simulink model "networkanalyzer"  (R2012b)
settings: Solver=ode3  SolverMode=SingleTasking  StartTime=0.0  StopTime=50000  RelTol=1e-3
libraries: xbsIndex_r4 x1097, casper_library_flow_control x33, casper_library_misc x21, xps_library x10
(part 3 of 8)

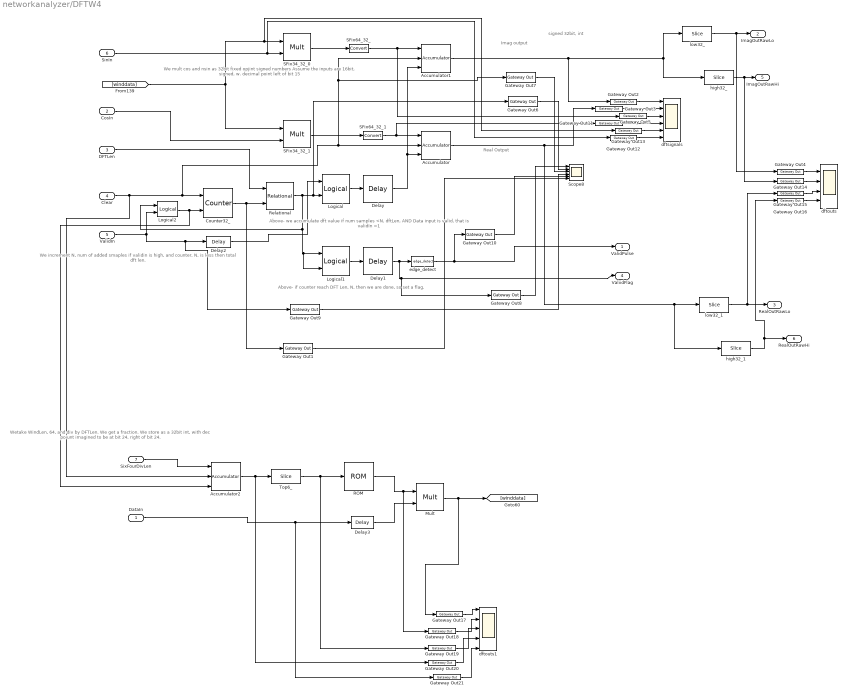
== system networkanalyzer/DFTW4 ==
  note: Wetake WindLen, 64, and div by DFTLen.
      | We get a fraction. We store as a 32bit int, with dec poiunt imagined to
      | be at bit 24, right of bit 24.
  note: Real Output
  note: Imag output
  note: We mult cos and nsin as 32bit fixed opjint signed numbers
      | Assume the inputs are 16bit, signed, w. decimal point left of bit 15
  note: Above- if counter reach DFT Len, N, then we are done, so set a flag.
  note: Above- we accumulate dft value if num samples <N, dftLen, AND
      | Data input is valid, that is validIn =1
  note: We increment N, num of added smaples if validin is high, and
      | counter, N, is less then total dft len.
  note: signed 32bit, int
  DataIn : Inport
  CosIn : Inport  Port=2
  DFTLen : Inport  Port=3
  Clear : Inport  Port=4
  ValidIn : Inport  Port=5
  SinIn : Inport  Port=6
  SixFourDivLen : Inport  Port=7
  Accumulator : xbsIndex_r4/Accumulator  operation=Add  n_bits=64  overflow=Wrap  scale=1  rst=on  hasbypass=off  en=on  dbl_ovrd=off  use_behavioral_HDL=on  implementation=Fabric  block_type=accum
  Accumulator1 : xbsIndex_r4/Accumulator  operation=Add  n_bits=64  overflow=Wrap  scale=1  rst=on  hasbypass=off  en=on  dbl_ovrd=off  use_behavioral_HDL=on  implementation=Fabric  block_type=accum
  Accumulator2 : xbsIndex_r4/Accumulator  operation=Add  n_bits=32  overflow=Wrap  scale=1  rst=on  hasbypass=off  en=on  dbl_ovrd=off  use_behavioral_HDL=on  implementation=Fabric  block_type=accum
  Counter32_ : xbsIndex_r4/Counter  cnt_type=Free Running  cnt_to=Inf  operation=Up  start_count=0  cnt_by_val=1  arith_type=Unsigned  n_bits=32  bin_pt=0  load_pin=off  rst=on  en=on  explicit_period=on  period=1  dbl_ovrd=off  use_behavioral_HDL=off  implementation=Fabric  block_type=counter
  Delay : xbsIndex_r4/Delay  rst=off  infoeditControl=Selection of Reset will increase slice count due to use of real FFs and instead of SRLs  en=off  latency=2  dbl_ovrd=off  reg_retiming=off  block_type=delay
  Delay1 : xbsIndex_r4/Delay  rst=off  infoeditControl=Selection of Reset will increase slice count due to use of real FFs and instead of SRLs  en=off  latency=2  dbl_ovrd=off  reg_retiming=off  block_type=delay
  Delay2 : xbsIndex_r4/Delay  rst=off  infoeditControl=Selection of Reset will increase slice count due to use of real FFs and instead of SRLs  en=off  latency=2  dbl_ovrd=off  reg_retiming=off  block_type=delay
  Delay3 : xbsIndex_r4/Delay  rst=off  infoeditControl=Selection of Reset will increase slice count due to use of real FFs and instead of SRLs  en=off  latency=1  dbl_ovrd=off  reg_retiming=off  block_type=delay
  Gateway Out{1..21} (21 alike) : xbsIndex_r4/Gateway Out  inherit_from_input=off  hdl_port=off  timing_constraint=None  locs_specified=off  LOCs={}  UseAsDAC=off  DACChannel='1'  block_type=gatewayout
  Logical : xbsIndex_r4/Logical  logical_function=AND  inputs=2  en=off  latency=1  precision=Full  arith_type=Unsigned  n_bits=16  bin_pt=0  align_bp=on  dbl_ovrd=off  block_type=logical
  Logical1 : xbsIndex_r4/Logical  logical_function=NAND  inputs=2  en=off  latency=1  precision=Full  arith_type=Unsigned  n_bits=16  bin_pt=0  align_bp=on  dbl_ovrd=off  block_type=logical
  Logical2 : xbsIndex_r4/Logical  logical_function=AND  inputs=2  en=off  latency=0  precision=Full  arith_type=Unsigned  n_bits=16  bin_pt=0  align_bp=on  dbl_ovrd=off  block_type=logical
  Mult : xbsIndex_r4/Mult  precision=User Defined  arith_type="Signed  (2's comp)"  n_bits=16  bin_pt=15  quantization=Truncate  overflow=Wrap  en=off  latency=3  dbl_ovrd=off  use_behavioral_HDL=off  opt=Speed  use_embedded=on  optimum_pipeline=off  pipeline=on  use_rpm=on  placement_style=Triangular  block_type=mult
  ROM : xbsIndex_r4/ROM  depth=64  initVector=0.5-0.5*cos(2*pi*(0:63)/63)  distributed_mem=Block RAM  rst=off  init_reg=0  en=off  latency=1  gui_display_data_type=Fixed-point  arith_type="Signed  (2's comp)"  n_bits=16  bin_pt=15  preci_type=Single  exp_width=8  frac_width=24  dbl_ovrd=off  optimize=Area  use_rpm=on  block_type=sprom
  Relational : xbsIndex_r4/Relational  mode=a>=b  en=off  latency=1  dbl_ovrd=off  block_type=relational
  SFix34_32_0 : xbsIndex_r4/Mult  precision=User Defined  arith_type="Signed  (2's comp)"  n_bits=34  bin_pt=32  quantization=Truncate  overflow=Saturate  en=off  latency=4  dbl_ovrd=off  use_behavioral_HDL=off  opt=Speed  use_embedded=on  optimum_pipeline=off  pipeline=on  use_rpm=on  placement_style=Triangular  block_type=mult
  SFix34_32_1 : xbsIndex_r4/Mult  precision=User Defined  arith_type="Signed  (2's comp)"  n_bits=34  bin_pt=32  quantization=Truncate  overflow=Saturate  en=off  latency=4  dbl_ovrd=off  use_behavioral_HDL=off  opt=Speed  use_embedded=on  optimum_pipeline=off  pipeline=on  use_rpm=on  placement_style=Triangular  block_type=mult
  SFix64_32_ : xbsIndex_r4/Convert  gui_display_data_type=Fixed-point  arith_type="Signed  (2's comp)"  n_bits=64  bin_pt=32  float_type=Single  exp_bits=8  fraction_bits=24  quantization=Truncate  overflow=Wrap  en=off  latency=0  dbl_ovrd=off  pipeline=off  block_type=convert
  SFix64_32_1 : xbsIndex_r4/Convert  gui_display_data_type=Fixed-point  arith_type="Signed  (2's comp)"  n_bits=64  bin_pt=32  float_type=Single  exp_bits=8  fraction_bits=24  quantization=Truncate  overflow=Wrap  en=off  latency=0  dbl_ovrd=off  pipeline=off  block_type=convert
  Scope8 : Scope  NumInputPorts=6
      settings: YMin=0~-5~-5~-5~-5~-5  YMax=300000~5~5~5~5~5  SaveName=ScopeData18  MaxDataPoints=10000
  Top6_ : xbsIndex_r4/Slice  nbits=6  boolean_output=off  mode=Upper Bit Location + Width  bit1=0  base1=MSB of Input  bit0=0  base0=LSB of Input  dbl_ovrd=off  block_type=slice
  dftouts : Scope  NumInputPorts=4
      settings: YMin=0~-5~-5~-5  YMax=300000~5~5~5  SaveName=ScopeData5  MaxDataPoints=10000
  dftouts1 : Scope  NumInputPorts=5
      settings: YMin=-1~0~0~0~-1  YMax=5.55112e-17~1~70~5e+09~0  MaxDataPoints=10000
  dftsignals : Scope  NumInputPorts=6
      settings: YMin=0~-5~-5~-5~-5~-5  YMax=300000~5~5~5~5~5  SaveName=ScopeData4  MaxDataPoints=10000
  edge_detect : casper_library_misc/edge_detect  edge=Rising  polarity=Active High  x_in=[0 0.08 0.08 0.16 0.16 0.24 0.24 0.32 0.32 0.4]  y_in="[-1 -1  1  1  1  1  1  1  1  1]"  x_out=[0.6 0.68 0.68 0.76 0.76 0.84 0.84 0.92 0.92 1]  y_out="[-1 -1  1  1 -1 -1 -1 -1 -1 -1]"
  high32_ : xbsIndex_r4/Slice  nbits=32  boolean_output=off  mode=Lower Bit Location + Width  bit1=-32  base1=MSB of Input  bit0=32  base0=LSB of Input  dbl_ovrd=off  block_type=slice
  high32_1 : xbsIndex_r4/Slice  nbits=32  boolean_output=off  mode=Lower Bit Location + Width  bit1=-31  base1=MSB of Input  bit0=32  base0=LSB of Input  dbl_ovrd=off  block_type=slice
  low32_ : xbsIndex_r4/Slice  nbits=32  boolean_output=off  mode=Lower Bit Location + Width  bit1=-31  base1=MSB of Input  bit0=0  base0=LSB of Input  dbl_ovrd=off  block_type=slice
  low32_1 : xbsIndex_r4/Slice  nbits=32  boolean_output=off  mode=Lower Bit Location + Width  bit1=-31  base1=MSB of Input  bit0=0  base0=LSB of Input  dbl_ovrd=off  block_type=slice
  ValidPulse : Outport
  ImagOutRawLo : Outport  Port=2
  RealOutRawLo : Outport  Port=3
  ValiidFlag : Outport  Port=4
  ImagOutRawHi : Outport  Port=5
  RealOutRawHi : Outport  Port=6
  wires:
  SFix34_32_1/1 -> SFix64_32_1/1
  Relational/1 -> Logical2/1, Logical1/2, Logical1/1, Gateway Out6/1, Logical/2
  Counter32_/1 -> Gateway Out1/1, Relational/2
  [winddata] -> SFix34_32_1/1, Gateway Out13/1, SFix34_32_0/1
  CosIn/1 -> SFix34_32_1/2
  DFTLen/1 -> Relational/1
  ValidIn/1 -> Logical2/2, Gateway Out9/1, Delay2/1
  Clear/1 -> Accumulator2/2, Gateway Out7/1, Accumulator1/2, Accumulator/2, Counter32_/1
  SinIn/1 -> Gateway Out12/1, SFix34_32_0/2
  Logical/1 -> Delay/1
  Delay/1 -> Accumulator1/3, Accumulator/3
  Logical1/1 -> Delay1/1
  Delay1/1 -> Gateway Out8/1, ValiidFlag/1, edge_detect/1
  edge_detect/1 -> Gateway Out10/1, ValidPulse/1
  Gateway Out6/1 -> Scope8/2
  Gateway Out7/1 -> Scope8/3
  Gateway Out8/1 -> Scope8/1
  Gateway Out9/1 -> Scope8/4
  Gateway Out10/1 -> Scope8/5
  Gateway Out1/1 -> Scope8/6
  Logical2/1 -> Accumulator2/3, Counter32_/2
  Delay2/1 -> Logical/1
  SFix34_32_0/1 -> SFix64_32_/1
  Gateway Out2/1 -> dftsignals/1
  Gateway Out3/1 -> dftsignals/2
  Gateway Out5/1 -> dftsignals/3
  Gateway Out13/1 -> dftsignals/5
  Gateway Out11/1 -> dftsignals/4
  Gateway Out12/1 -> dftsignals/6
  SFix64_32_/1 -> Gateway Out5/1, Accumulator1/1
  SFix64_32_1/1 -> Gateway Out11/1, Accumulator/1
  Accumulator1/1 -> Gateway Out2/1, high32_/1, low32_/1
  Accumulator/1 -> high32_1/1, low32_1/1, Gateway Out3/1
  low32_/1 -> Gateway Out4/1, ImagOutRawLo/1
  high32_/1 -> Gateway Out14/1, ImagOutRawHi/1
  low32_1/1 -> Gateway Out15/1, RealOutRawLo/1
  high32_1/1 -> Gateway Out16/1, RealOutRawHi/1
  Gateway Out15/1 -> dftouts/3
  Gateway Out16/1 -> dftouts/4
  Gateway Out14/1 -> dftouts/2
  Gateway Out4/1 -> dftouts/1
  ROM/1 -> Gateway Out18/1, Mult/1
  Delay3/1 -> Mult/2
  Mult/1 -> Gateway Out17/1, [winddata]
  Top6_/1 -> Gateway Out19/1, ROM/1
  Accumulator2/1 -> Gateway Out20/1, Top6_/1
  SixFourDivLen/1 -> Accumulator2/1
  DataIn/1 -> Gateway Out21/1, Delay3/1
  Gateway Out17/1 -> dftouts1/1
  Gateway Out18/1 -> dftouts1/2
  Gateway Out19/1 -> dftouts1/3
  Gateway Out20/1 -> dftouts1/4
  Gateway Out21/1 -> dftouts1/5

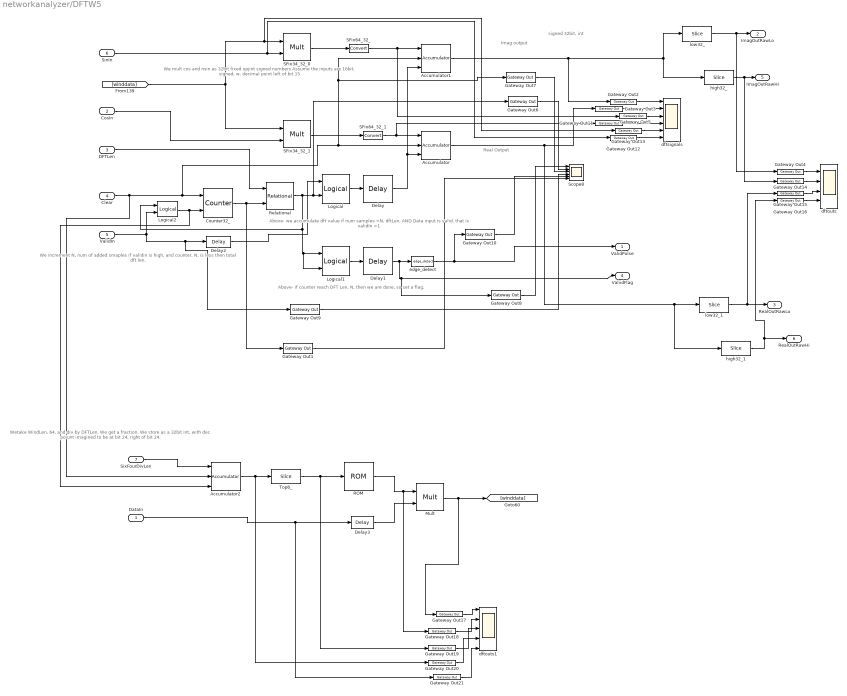
== system networkanalyzer/DFTW5 ==
  note: Wetake WindLen, 64, and div by DFTLen.
      | We get a fraction. We store as a 32bit int, with dec poiunt imagined to
      | be at bit 24, right of bit 24.
  note: Real Output
  note: Imag output
  note: We mult cos and nsin as 32bit fixed opjint signed numbers
      | Assume the inputs are 16bit, signed, w. decimal point left of bit 15
  note: Above- if counter reach DFT Len, N, then we are done, so set a flag.
  note: Above- we accumulate dft value if num samples <N, dftLen, AND
      | Data input is valid, that is validIn =1
  note: We increment N, num of added smaples if validin is high, and
      | counter, N, is less then total dft len.
  note: signed 32bit, int
  DataIn : Inport
  CosIn : Inport  Port=2
  DFTLen : Inport  Port=3
  Clear : Inport  Port=4
  ValidIn : Inport  Port=5
  SinIn : Inport  Port=6
  SixFourDivLen : Inport  Port=7
  Accumulator : xbsIndex_r4/Accumulator  operation=Add  n_bits=64  overflow=Wrap  scale=1  rst=on  hasbypass=off  en=on  dbl_ovrd=off  use_behavioral_HDL=on  implementation=Fabric  block_type=accum
  Accumulator1 : xbsIndex_r4/Accumulator  operation=Add  n_bits=64  overflow=Wrap  scale=1  rst=on  hasbypass=off  en=on  dbl_ovrd=off  use_behavioral_HDL=on  implementation=Fabric  block_type=accum
  Accumulator2 : xbsIndex_r4/Accumulator  operation=Add  n_bits=32  overflow=Wrap  scale=1  rst=on  hasbypass=off  en=on  dbl_ovrd=off  use_behavioral_HDL=on  implementation=Fabric  block_type=accum
  Counter32_ : xbsIndex_r4/Counter  cnt_type=Free Running  cnt_to=Inf  operation=Up  start_count=0  cnt_by_val=1  arith_type=Unsigned  n_bits=32  bin_pt=0  load_pin=off  rst=on  en=on  explicit_period=on  period=1  dbl_ovrd=off  use_behavioral_HDL=off  implementation=Fabric  block_type=counter
  Delay : xbsIndex_r4/Delay  rst=off  infoeditControl=Selection of Reset will increase slice count due to use of real FFs and instead of SRLs  en=off  latency=2  dbl_ovrd=off  reg_retiming=off  block_type=delay
  Delay1 : xbsIndex_r4/Delay  rst=off  infoeditControl=Selection of Reset will increase slice count due to use of real FFs and instead of SRLs  en=off  latency=2  dbl_ovrd=off  reg_retiming=off  block_type=delay
  Delay2 : xbsIndex_r4/Delay  rst=off  infoeditControl=Selection of Reset will increase slice count due to use of real FFs and instead of SRLs  en=off  latency=2  dbl_ovrd=off  reg_retiming=off  block_type=delay
  Delay3 : xbsIndex_r4/Delay  rst=off  infoeditControl=Selection of Reset will increase slice count due to use of real FFs and instead of SRLs  en=off  latency=1  dbl_ovrd=off  reg_retiming=off  block_type=delay
  Gateway Out{1..21} (21 alike) : xbsIndex_r4/Gateway Out  inherit_from_input=off  hdl_port=off  timing_constraint=None  locs_specified=off  LOCs={}  UseAsDAC=off  DACChannel='1'  block_type=gatewayout
  Logical : xbsIndex_r4/Logical  logical_function=AND  inputs=2  en=off  latency=1  precision=Full  arith_type=Unsigned  n_bits=16  bin_pt=0  align_bp=on  dbl_ovrd=off  block_type=logical
  Logical1 : xbsIndex_r4/Logical  logical_function=NAND  inputs=2  en=off  latency=1  precision=Full  arith_type=Unsigned  n_bits=16  bin_pt=0  align_bp=on  dbl_ovrd=off  block_type=logical
  Logical2 : xbsIndex_r4/Logical  logical_function=AND  inputs=2  en=off  latency=0  precision=Full  arith_type=Unsigned  n_bits=16  bin_pt=0  align_bp=on  dbl_ovrd=off  block_type=logical
  Mult : xbsIndex_r4/Mult  precision=User Defined  arith_type="Signed  (2's comp)"  n_bits=16  bin_pt=15  quantization=Truncate  overflow=Wrap  en=off  latency=3  dbl_ovrd=off  use_behavioral_HDL=off  opt=Speed  use_embedded=on  optimum_pipeline=off  pipeline=on  use_rpm=on  placement_style=Triangular  block_type=mult
  ROM : xbsIndex_r4/ROM  depth=64  initVector=0.5-0.5*cos(2*pi*(0:63)/63)  distributed_mem=Block RAM  rst=off  init_reg=0  en=off  latency=1  gui_display_data_type=Fixed-point  arith_type="Signed  (2's comp)"  n_bits=16  bin_pt=15  preci_type=Single  exp_width=8  frac_width=24  dbl_ovrd=off  optimize=Area  use_rpm=on  block_type=sprom
  Relational : xbsIndex_r4/Relational  mode=a>=b  en=off  latency=1  dbl_ovrd=off  block_type=relational
  SFix34_32_0 : xbsIndex_r4/Mult  precision=User Defined  arith_type="Signed  (2's comp)"  n_bits=34  bin_pt=32  quantization=Truncate  overflow=Saturate  en=off  latency=4  dbl_ovrd=off  use_behavioral_HDL=off  opt=Speed  use_embedded=on  optimum_pipeline=off  pipeline=on  use_rpm=on  placement_style=Triangular  block_type=mult
  SFix34_32_1 : xbsIndex_r4/Mult  precision=User Defined  arith_type="Signed  (2's comp)"  n_bits=34  bin_pt=32  quantization=Truncate  overflow=Saturate  en=off  latency=4  dbl_ovrd=off  use_behavioral_HDL=off  opt=Speed  use_embedded=on  optimum_pipeline=off  pipeline=on  use_rpm=on  placement_style=Triangular  block_type=mult
  SFix64_32_ : xbsIndex_r4/Convert  gui_display_data_type=Fixed-point  arith_type="Signed  (2's comp)"  n_bits=64  bin_pt=32  float_type=Single  exp_bits=8  fraction_bits=24  quantization=Truncate  overflow=Wrap  en=off  latency=0  dbl_ovrd=off  pipeline=off  block_type=convert
  SFix64_32_1 : xbsIndex_r4/Convert  gui_display_data_type=Fixed-point  arith_type="Signed  (2's comp)"  n_bits=64  bin_pt=32  float_type=Single  exp_bits=8  fraction_bits=24  quantization=Truncate  overflow=Wrap  en=off  latency=0  dbl_ovrd=off  pipeline=off  block_type=convert
  Scope8 : Scope  NumInputPorts=6
      settings: YMin=0~-5~-5~-5~-5~-5  YMax=300000~5~5~5~5~5  SaveName=ScopeData18  MaxDataPoints=10000
  Top6_ : xbsIndex_r4/Slice  nbits=6  boolean_output=off  mode=Upper Bit Location + Width  bit1=0  base1=MSB of Input  bit0=0  base0=LSB of Input  dbl_ovrd=off  block_type=slice
  dftouts : Scope  NumInputPorts=4
      settings: YMin=0~-5~-5~-5  YMax=300000~5~5~5  SaveName=ScopeData5  MaxDataPoints=10000
  dftouts1 : Scope  NumInputPorts=5
      settings: YMin=-1~0~0~0~-1  YMax=5.55112e-17~1~70~5e+09~0  MaxDataPoints=10000
  dftsignals : Scope  NumInputPorts=6
      settings: YMin=0~-5~-5~-5~-5~-5  YMax=300000~5~5~5~5~5  SaveName=ScopeData4  MaxDataPoints=10000
  edge_detect : casper_library_misc/edge_detect  edge=Rising  polarity=Active High  x_in=[0 0.08 0.08 0.16 0.16 0.24 0.24 0.32 0.32 0.4]  y_in="[-1 -1  1  1  1  1  1  1  1  1]"  x_out=[0.6 0.68 0.68 0.76 0.76 0.84 0.84 0.92 0.92 1]  y_out="[-1 -1  1  1 -1 -1 -1 -1 -1 -1]"
  high32_ : xbsIndex_r4/Slice  nbits=32  boolean_output=off  mode=Lower Bit Location + Width  bit1=-32  base1=MSB of Input  bit0=32  base0=LSB of Input  dbl_ovrd=off  block_type=slice
  high32_1 : xbsIndex_r4/Slice  nbits=32  boolean_output=off  mode=Lower Bit Location + Width  bit1=-31  base1=MSB of Input  bit0=32  base0=LSB of Input  dbl_ovrd=off  block_type=slice
  low32_ : xbsIndex_r4/Slice  nbits=32  boolean_output=off  mode=Lower Bit Location + Width  bit1=-31  base1=MSB of Input  bit0=0  base0=LSB of Input  dbl_ovrd=off  block_type=slice
  low32_1 : xbsIndex_r4/Slice  nbits=32  boolean_output=off  mode=Lower Bit Location + Width  bit1=-31  base1=MSB of Input  bit0=0  base0=LSB of Input  dbl_ovrd=off  block_type=slice
  ValidPulse : Outport
  ImagOutRawLo : Outport  Port=2
  RealOutRawLo : Outport  Port=3
  ValiidFlag : Outport  Port=4
  ImagOutRawHi : Outport  Port=5
  RealOutRawHi : Outport  Port=6
  wires:
  SFix34_32_1/1 -> SFix64_32_1/1
  Relational/1 -> Logical2/1, Logical1/2, Logical1/1, Gateway Out6/1, Logical/2
  Counter32_/1 -> Gateway Out1/1, Relational/2
  [winddata] -> SFix34_32_1/1, Gateway Out13/1, SFix34_32_0/1
  CosIn/1 -> SFix34_32_1/2
  DFTLen/1 -> Relational/1
  ValidIn/1 -> Logical2/2, Gateway Out9/1, Delay2/1
  Clear/1 -> Accumulator2/2, Gateway Out7/1, Accumulator1/2, Accumulator/2, Counter32_/1
  SinIn/1 -> Gateway Out12/1, SFix34_32_0/2
  Logical/1 -> Delay/1
  Delay/1 -> Accumulator1/3, Accumulator/3
  Logical1/1 -> Delay1/1
  Delay1/1 -> Gateway Out8/1, ValiidFlag/1, edge_detect/1
  edge_detect/1 -> Gateway Out10/1, ValidPulse/1
  Gateway Out6/1 -> Scope8/2
  Gateway Out7/1 -> Scope8/3
  Gateway Out8/1 -> Scope8/1
  Gateway Out9/1 -> Scope8/4
  Gateway Out10/1 -> Scope8/5
  Gateway Out1/1 -> Scope8/6
  Logical2/1 -> Accumulator2/3, Counter32_/2
  Delay2/1 -> Logical/1
  SFix34_32_0/1 -> SFix64_32_/1
  Gateway Out2/1 -> dftsignals/1
  Gateway Out3/1 -> dftsignals/2
  Gateway Out5/1 -> dftsignals/3
  Gateway Out13/1 -> dftsignals/5
  Gateway Out11/1 -> dftsignals/4
  Gateway Out12/1 -> dftsignals/6
  SFix64_32_/1 -> Gateway Out5/1, Accumulator1/1
  SFix64_32_1/1 -> Gateway Out11/1, Accumulator/1
  Accumulator1/1 -> Gateway Out2/1, high32_/1, low32_/1
  Accumulator/1 -> high32_1/1, low32_1/1, Gateway Out3/1
  low32_/1 -> Gateway Out4/1, ImagOutRawLo/1
  high32_/1 -> Gateway Out14/1, ImagOutRawHi/1
  low32_1/1 -> Gateway Out15/1, RealOutRawLo/1
  high32_1/1 -> Gateway Out16/1, RealOutRawHi/1
  Gateway Out15/1 -> dftouts/3
  Gateway Out16/1 -> dftouts/4
  Gateway Out14/1 -> dftouts/2
  Gateway Out4/1 -> dftouts/1
  ROM/1 -> Gateway Out18/1, Mult/1
  Delay3/1 -> Mult/2
  Mult/1 -> Gateway Out17/1, [winddata]
  Top6_/1 -> Gateway Out19/1, ROM/1
  Accumulator2/1 -> Gateway Out20/1, Top6_/1
  SixFourDivLen/1 -> Accumulator2/1
  DataIn/1 -> Gateway Out21/1, Delay3/1
  Gateway Out17/1 -> dftouts1/1
  Gateway Out18/1 -> dftouts1/2
  Gateway Out19/1 -> dftouts1/3
  Gateway Out20/1 -> dftouts1/4
  Gateway Out21/1 -> dftouts1/5

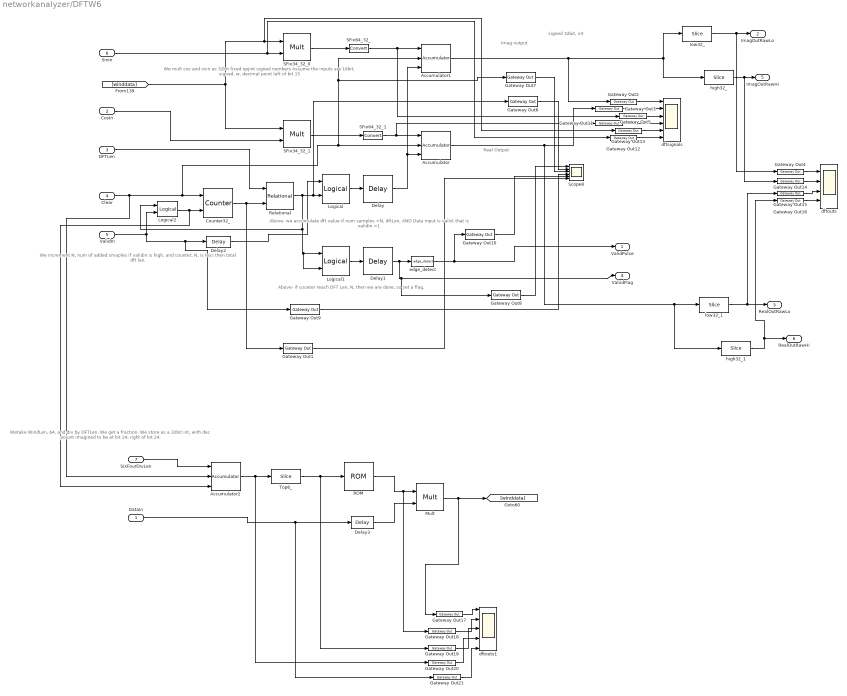
== system networkanalyzer/DFTW6 ==
  note: Wetake WindLen, 64, and div by DFTLen.
      | We get a fraction. We store as a 32bit int, with dec poiunt imagined to
      | be at bit 24, right of bit 24.
  note: Real Output
  note: Imag output
  note: We mult cos and nsin as 32bit fixed opjint signed numbers
      | Assume the inputs are 16bit, signed, w. decimal point left of bit 15
  note: Above- if counter reach DFT Len, N, then we are done, so set a flag.
  note: Above- we accumulate dft value if num samples <N, dftLen, AND
      | Data input is valid, that is validIn =1
  note: We increment N, num of added smaples if validin is high, and
      | counter, N, is less then total dft len.
  note: signed 32bit, int
  DataIn : Inport
  CosIn : Inport  Port=2
  DFTLen : Inport  Port=3
  Clear : Inport  Port=4
  ValidIn : Inport  Port=5
  SinIn : Inport  Port=6
  SixFourDivLen : Inport  Port=7
  Accumulator : xbsIndex_r4/Accumulator  operation=Add  n_bits=64  overflow=Wrap  scale=1  rst=on  hasbypass=off  en=on  dbl_ovrd=off  use_behavioral_HDL=on  implementation=Fabric  block_type=accum
  Accumulator1 : xbsIndex_r4/Accumulator  operation=Add  n_bits=64  overflow=Wrap  scale=1  rst=on  hasbypass=off  en=on  dbl_ovrd=off  use_behavioral_HDL=on  implementation=Fabric  block_type=accum
  Accumulator2 : xbsIndex_r4/Accumulator  operation=Add  n_bits=32  overflow=Wrap  scale=1  rst=on  hasbypass=off  en=on  dbl_ovrd=off  use_behavioral_HDL=on  implementation=Fabric  block_type=accum
  Counter32_ : xbsIndex_r4/Counter  cnt_type=Free Running  cnt_to=Inf  operation=Up  start_count=0  cnt_by_val=1  arith_type=Unsigned  n_bits=32  bin_pt=0  load_pin=off  rst=on  en=on  explicit_period=on  period=1  dbl_ovrd=off  use_behavioral_HDL=off  implementation=Fabric  block_type=counter
  Delay : xbsIndex_r4/Delay  rst=off  infoeditControl=Selection of Reset will increase slice count due to use of real FFs and instead of SRLs  en=off  latency=2  dbl_ovrd=off  reg_retiming=off  block_type=delay
  Delay1 : xbsIndex_r4/Delay  rst=off  infoeditControl=Selection of Reset will increase slice count due to use of real FFs and instead of SRLs  en=off  latency=2  dbl_ovrd=off  reg_retiming=off  block_type=delay
  Delay2 : xbsIndex_r4/Delay  rst=off  infoeditControl=Selection of Reset will increase slice count due to use of real FFs and instead of SRLs  en=off  latency=2  dbl_ovrd=off  reg_retiming=off  block_type=delay
  Delay3 : xbsIndex_r4/Delay  rst=off  infoeditControl=Selection of Reset will increase slice count due to use of real FFs and instead of SRLs  en=off  latency=1  dbl_ovrd=off  reg_retiming=off  block_type=delay
  Gateway Out{1..21} (21 alike) : xbsIndex_r4/Gateway Out  inherit_from_input=off  hdl_port=off  timing_constraint=None  locs_specified=off  LOCs={}  UseAsDAC=off  DACChannel='1'  block_type=gatewayout
  Logical : xbsIndex_r4/Logical  logical_function=AND  inputs=2  en=off  latency=1  precision=Full  arith_type=Unsigned  n_bits=16  bin_pt=0  align_bp=on  dbl_ovrd=off  block_type=logical
  Logical1 : xbsIndex_r4/Logical  logical_function=NAND  inputs=2  en=off  latency=1  precision=Full  arith_type=Unsigned  n_bits=16  bin_pt=0  align_bp=on  dbl_ovrd=off  block_type=logical
  Logical2 : xbsIndex_r4/Logical  logical_function=AND  inputs=2  en=off  latency=0  precision=Full  arith_type=Unsigned  n_bits=16  bin_pt=0  align_bp=on  dbl_ovrd=off  block_type=logical
  Mult : xbsIndex_r4/Mult  precision=User Defined  arith_type="Signed  (2's comp)"  n_bits=16  bin_pt=15  quantization=Truncate  overflow=Wrap  en=off  latency=3  dbl_ovrd=off  use_behavioral_HDL=off  opt=Speed  use_embedded=on  optimum_pipeline=off  pipeline=on  use_rpm=on  placement_style=Triangular  block_type=mult
  ROM : xbsIndex_r4/ROM  depth=64  initVector=0.5-0.5*cos(2*pi*(0:63)/63)  distributed_mem=Block RAM  rst=off  init_reg=0  en=off  latency=1  gui_display_data_type=Fixed-point  arith_type="Signed  (2's comp)"  n_bits=16  bin_pt=15  preci_type=Single  exp_width=8  frac_width=24  dbl_ovrd=off  optimize=Area  use_rpm=on  block_type=sprom
  Relational : xbsIndex_r4/Relational  mode=a>=b  en=off  latency=1  dbl_ovrd=off  block_type=relational
  SFix34_32_0 : xbsIndex_r4/Mult  precision=User Defined  arith_type="Signed  (2's comp)"  n_bits=34  bin_pt=32  quantization=Truncate  overflow=Saturate  en=off  latency=4  dbl_ovrd=off  use_behavioral_HDL=off  opt=Speed  use_embedded=on  optimum_pipeline=off  pipeline=on  use_rpm=on  placement_style=Triangular  block_type=mult
  SFix34_32_1 : xbsIndex_r4/Mult  precision=User Defined  arith_type="Signed  (2's comp)"  n_bits=34  bin_pt=32  quantization=Truncate  overflow=Saturate  en=off  latency=4  dbl_ovrd=off  use_behavioral_HDL=off  opt=Speed  use_embedded=on  optimum_pipeline=off  pipeline=on  use_rpm=on  placement_style=Triangular  block_type=mult
  SFix64_32_ : xbsIndex_r4/Convert  gui_display_data_type=Fixed-point  arith_type="Signed  (2's comp)"  n_bits=64  bin_pt=32  float_type=Single  exp_bits=8  fraction_bits=24  quantization=Truncate  overflow=Wrap  en=off  latency=0  dbl_ovrd=off  pipeline=off  block_type=convert
  SFix64_32_1 : xbsIndex_r4/Convert  gui_display_data_type=Fixed-point  arith_type="Signed  (2's comp)"  n_bits=64  bin_pt=32  float_type=Single  exp_bits=8  fraction_bits=24  quantization=Truncate  overflow=Wrap  en=off  latency=0  dbl_ovrd=off  pipeline=off  block_type=convert
  Scope8 : Scope  NumInputPorts=6
      settings: YMin=0~-5~-5~-5~-5~-5  YMax=300000~5~5~5~5~5  SaveName=ScopeData18  MaxDataPoints=10000
  Top6_ : xbsIndex_r4/Slice  nbits=6  boolean_output=off  mode=Upper Bit Location + Width  bit1=0  base1=MSB of Input  bit0=0  base0=LSB of Input  dbl_ovrd=off  block_type=slice
  dftouts : Scope  NumInputPorts=4
      settings: YMin=0~-5~-5~-5  YMax=300000~5~5~5  SaveName=ScopeData5  MaxDataPoints=10000
  dftouts1 : Scope  NumInputPorts=5
      settings: YMin=-1~0~0~0~-1  YMax=5.55112e-17~1~70~5e+09~0  MaxDataPoints=10000
  dftsignals : Scope  NumInputPorts=6
      settings: YMin=0~-5~-5~-5~-5~-5  YMax=300000~5~5~5~5~5  SaveName=ScopeData4  MaxDataPoints=10000
  edge_detect : casper_library_misc/edge_detect  edge=Rising  polarity=Active High  x_in=[0 0.08 0.08 0.16 0.16 0.24 0.24 0.32 0.32 0.4]  y_in="[-1 -1  1  1  1  1  1  1  1  1]"  x_out=[0.6 0.68 0.68 0.76 0.76 0.84 0.84 0.92 0.92 1]  y_out="[-1 -1  1  1 -1 -1 -1 -1 -1 -1]"
  high32_ : xbsIndex_r4/Slice  nbits=32  boolean_output=off  mode=Lower Bit Location + Width  bit1=-32  base1=MSB of Input  bit0=32  base0=LSB of Input  dbl_ovrd=off  block_type=slice
  high32_1 : xbsIndex_r4/Slice  nbits=32  boolean_output=off  mode=Lower Bit Location + Width  bit1=-31  base1=MSB of Input  bit0=32  base0=LSB of Input  dbl_ovrd=off  block_type=slice
  low32_ : xbsIndex_r4/Slice  nbits=32  boolean_output=off  mode=Lower Bit Location + Width  bit1=-31  base1=MSB of Input  bit0=0  base0=LSB of Input  dbl_ovrd=off  block_type=slice
  low32_1 : xbsIndex_r4/Slice  nbits=32  boolean_output=off  mode=Lower Bit Location + Width  bit1=-31  base1=MSB of Input  bit0=0  base0=LSB of Input  dbl_ovrd=off  block_type=slice
  ValidPulse : Outport
  ImagOutRawLo : Outport  Port=2
  RealOutRawLo : Outport  Port=3
  ValiidFlag : Outport  Port=4
  ImagOutRawHi : Outport  Port=5
  RealOutRawHi : Outport  Port=6
  wires:
  SFix34_32_1/1 -> SFix64_32_1/1
  Relational/1 -> Logical2/1, Logical1/2, Logical1/1, Gateway Out6/1, Logical/2
  Counter32_/1 -> Gateway Out1/1, Relational/2
  [winddata] -> SFix34_32_1/1, Gateway Out13/1, SFix34_32_0/1
  CosIn/1 -> SFix34_32_1/2
  DFTLen/1 -> Relational/1
  ValidIn/1 -> Logical2/2, Gateway Out9/1, Delay2/1
  Clear/1 -> Accumulator2/2, Gateway Out7/1, Accumulator1/2, Accumulator/2, Counter32_/1
  SinIn/1 -> Gateway Out12/1, SFix34_32_0/2
  Logical/1 -> Delay/1
  Delay/1 -> Accumulator1/3, Accumulator/3
  Logical1/1 -> Delay1/1
  Delay1/1 -> Gateway Out8/1, ValiidFlag/1, edge_detect/1
  edge_detect/1 -> Gateway Out10/1, ValidPulse/1
  Gateway Out6/1 -> Scope8/2
  Gateway Out7/1 -> Scope8/3
  Gateway Out8/1 -> Scope8/1
  Gateway Out9/1 -> Scope8/4
  Gateway Out10/1 -> Scope8/5
  Gateway Out1/1 -> Scope8/6
  Logical2/1 -> Accumulator2/3, Counter32_/2
  Delay2/1 -> Logical/1
  SFix34_32_0/1 -> SFix64_32_/1
  Gateway Out2/1 -> dftsignals/1
  Gateway Out3/1 -> dftsignals/2
  Gateway Out5/1 -> dftsignals/3
  Gateway Out13/1 -> dftsignals/5
  Gateway Out11/1 -> dftsignals/4
  Gateway Out12/1 -> dftsignals/6
  SFix64_32_/1 -> Gateway Out5/1, Accumulator1/1
  SFix64_32_1/1 -> Gateway Out11/1, Accumulator/1
  Accumulator1/1 -> Gateway Out2/1, high32_/1, low32_/1
  Accumulator/1 -> high32_1/1, low32_1/1, Gateway Out3/1
  low32_/1 -> Gateway Out4/1, ImagOutRawLo/1
  high32_/1 -> Gateway Out14/1, ImagOutRawHi/1
  low32_1/1 -> Gateway Out15/1, RealOutRawLo/1
  high32_1/1 -> Gateway Out16/1, RealOutRawHi/1
  Gateway Out15/1 -> dftouts/3
  Gateway Out16/1 -> dftouts/4
  Gateway Out14/1 -> dftouts/2
  Gateway Out4/1 -> dftouts/1
  ROM/1 -> Gateway Out18/1, Mult/1
  Delay3/1 -> Mult/2
  Mult/1 -> Gateway Out17/1, [winddata]
  Top6_/1 -> Gateway Out19/1, ROM/1
  Accumulator2/1 -> Gateway Out20/1, Top6_/1
  SixFourDivLen/1 -> Accumulator2/1
  DataIn/1 -> Gateway Out21/1, Delay3/1
  Gateway Out17/1 -> dftouts1/1
  Gateway Out18/1 -> dftouts1/2
  Gateway Out19/1 -> dftouts1/3
  Gateway Out20/1 -> dftouts1/4
  Gateway Out21/1 -> dftouts1/5

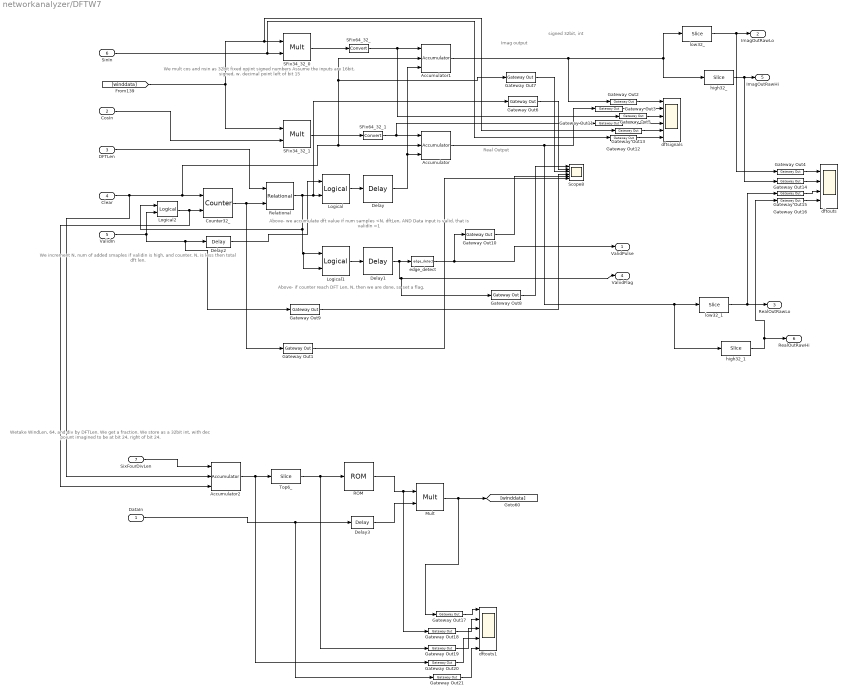
== system networkanalyzer/DFTW7 ==
  note: Wetake WindLen, 64, and div by DFTLen.
      | We get a fraction. We store as a 32bit int, with dec poiunt imagined to
      | be at bit 24, right of bit 24.
  note: Real Output
  note: Imag output
  note: We mult cos and nsin as 32bit fixed opjint signed numbers
      | Assume the inputs are 16bit, signed, w. decimal point left of bit 15
  note: Above- if counter reach DFT Len, N, then we are done, so set a flag.
  note: Above- we accumulate dft value if num samples <N, dftLen, AND
      | Data input is valid, that is validIn =1
  note: We increment N, num of added smaples if validin is high, and
      | counter, N, is less then total dft len.
  note: signed 32bit, int
  DataIn : Inport
  CosIn : Inport  Port=2
  DFTLen : Inport  Port=3
  Clear : Inport  Port=4
  ValidIn : Inport  Port=5
  SinIn : Inport  Port=6
  SixFourDivLen : Inport  Port=7
  Accumulator : xbsIndex_r4/Accumulator  operation=Add  n_bits=64  overflow=Wrap  scale=1  rst=on  hasbypass=off  en=on  dbl_ovrd=off  use_behavioral_HDL=on  implementation=Fabric  block_type=accum
  Accumulator1 : xbsIndex_r4/Accumulator  operation=Add  n_bits=64  overflow=Wrap  scale=1  rst=on  hasbypass=off  en=on  dbl_ovrd=off  use_behavioral_HDL=on  implementation=Fabric  block_type=accum
  Accumulator2 : xbsIndex_r4/Accumulator  operation=Add  n_bits=32  overflow=Wrap  scale=1  rst=on  hasbypass=off  en=on  dbl_ovrd=off  use_behavioral_HDL=on  implementation=Fabric  block_type=accum
  Counter32_ : xbsIndex_r4/Counter  cnt_type=Free Running  cnt_to=Inf  operation=Up  start_count=0  cnt_by_val=1  arith_type=Unsigned  n_bits=32  bin_pt=0  load_pin=off  rst=on  en=on  explicit_period=on  period=1  dbl_ovrd=off  use_behavioral_HDL=off  implementation=Fabric  block_type=counter
  Delay : xbsIndex_r4/Delay  rst=off  infoeditControl=Selection of Reset will increase slice count due to use of real FFs and instead of SRLs  en=off  latency=2  dbl_ovrd=off  reg_retiming=off  block_type=delay
  Delay1 : xbsIndex_r4/Delay  rst=off  infoeditControl=Selection of Reset will increase slice count due to use of real FFs and instead of SRLs  en=off  latency=2  dbl_ovrd=off  reg_retiming=off  block_type=delay
  Delay2 : xbsIndex_r4/Delay  rst=off  infoeditControl=Selection of Reset will increase slice count due to use of real FFs and instead of SRLs  en=off  latency=2  dbl_ovrd=off  reg_retiming=off  block_type=delay
  Delay3 : xbsIndex_r4/Delay  rst=off  infoeditControl=Selection of Reset will increase slice count due to use of real FFs and instead of SRLs  en=off  latency=1  dbl_ovrd=off  reg_retiming=off  block_type=delay
  Gateway Out{1..21} (21 alike) : xbsIndex_r4/Gateway Out  inherit_from_input=off  hdl_port=off  timing_constraint=None  locs_specified=off  LOCs={}  UseAsDAC=off  DACChannel='1'  block_type=gatewayout
  Logical : xbsIndex_r4/Logical  logical_function=AND  inputs=2  en=off  latency=1  precision=Full  arith_type=Unsigned  n_bits=16  bin_pt=0  align_bp=on  dbl_ovrd=off  block_type=logical
  Logical1 : xbsIndex_r4/Logical  logical_function=NAND  inputs=2  en=off  latency=1  precision=Full  arith_type=Unsigned  n_bits=16  bin_pt=0  align_bp=on  dbl_ovrd=off  block_type=logical
  Logical2 : xbsIndex_r4/Logical  logical_function=AND  inputs=2  en=off  latency=0  precision=Full  arith_type=Unsigned  n_bits=16  bin_pt=0  align_bp=on  dbl_ovrd=off  block_type=logical
  Mult : xbsIndex_r4/Mult  precision=User Defined  arith_type="Signed  (2's comp)"  n_bits=16  bin_pt=15  quantization=Truncate  overflow=Wrap  en=off  latency=3  dbl_ovrd=off  use_behavioral_HDL=off  opt=Speed  use_embedded=on  optimum_pipeline=off  pipeline=on  use_rpm=on  placement_style=Triangular  block_type=mult
  ROM : xbsIndex_r4/ROM  depth=64  initVector=0.5-0.5*cos(2*pi*(0:63)/63)  distributed_mem=Block RAM  rst=off  init_reg=0  en=off  latency=1  gui_display_data_type=Fixed-point  arith_type="Signed  (2's comp)"  n_bits=16  bin_pt=15  preci_type=Single  exp_width=8  frac_width=24  dbl_ovrd=off  optimize=Area  use_rpm=on  block_type=sprom
  Relational : xbsIndex_r4/Relational  mode=a>=b  en=off  latency=1  dbl_ovrd=off  block_type=relational
  SFix34_32_0 : xbsIndex_r4/Mult  precision=User Defined  arith_type="Signed  (2's comp)"  n_bits=34  bin_pt=32  quantization=Truncate  overflow=Saturate  en=off  latency=4  dbl_ovrd=off  use_behavioral_HDL=off  opt=Speed  use_embedded=on  optimum_pipeline=off  pipeline=on  use_rpm=on  placement_style=Triangular  block_type=mult
  SFix34_32_1 : xbsIndex_r4/Mult  precision=User Defined  arith_type="Signed  (2's comp)"  n_bits=34  bin_pt=32  quantization=Truncate  overflow=Saturate  en=off  latency=4  dbl_ovrd=off  use_behavioral_HDL=off  opt=Speed  use_embedded=on  optimum_pipeline=off  pipeline=on  use_rpm=on  placement_style=Triangular  block_type=mult
  SFix64_32_ : xbsIndex_r4/Convert  gui_display_data_type=Fixed-point  arith_type="Signed  (2's comp)"  n_bits=64  bin_pt=32  float_type=Single  exp_bits=8  fraction_bits=24  quantization=Truncate  overflow=Wrap  en=off  latency=0  dbl_ovrd=off  pipeline=off  block_type=convert
  SFix64_32_1 : xbsIndex_r4/Convert  gui_display_data_type=Fixed-point  arith_type="Signed  (2's comp)"  n_bits=64  bin_pt=32  float_type=Single  exp_bits=8  fraction_bits=24  quantization=Truncate  overflow=Wrap  en=off  latency=0  dbl_ovrd=off  pipeline=off  block_type=convert
  Scope8 : Scope  NumInputPorts=6
      settings: YMin=0~-5~-5~-5~-5~-5  YMax=300000~5~5~5~5~5  SaveName=ScopeData18  MaxDataPoints=10000
  Top6_ : xbsIndex_r4/Slice  nbits=6  boolean_output=off  mode=Upper Bit Location + Width  bit1=0  base1=MSB of Input  bit0=0  base0=LSB of Input  dbl_ovrd=off  block_type=slice
  dftouts : Scope  NumInputPorts=4
      settings: YMin=0~-5~-5~-5  YMax=300000~5~5~5  SaveName=ScopeData5  MaxDataPoints=10000
  dftouts1 : Scope  NumInputPorts=5
      settings: YMin=-1~0~0~0~-1  YMax=5.55112e-17~1~70~5e+09~0  MaxDataPoints=10000
  dftsignals : Scope  NumInputPorts=6
      settings: YMin=0~-5~-5~-5~-5~-5  YMax=300000~5~5~5~5~5  SaveName=ScopeData4  MaxDataPoints=10000
  edge_detect : casper_library_misc/edge_detect  edge=Rising  polarity=Active High  x_in=[0 0.08 0.08 0.16 0.16 0.24 0.24 0.32 0.32 0.4]  y_in="[-1 -1  1  1  1  1  1  1  1  1]"  x_out=[0.6 0.68 0.68 0.76 0.76 0.84 0.84 0.92 0.92 1]  y_out="[-1 -1  1  1 -1 -1 -1 -1 -1 -1]"
  high32_ : xbsIndex_r4/Slice  nbits=32  boolean_output=off  mode=Lower Bit Location + Width  bit1=-32  base1=MSB of Input  bit0=32  base0=LSB of Input  dbl_ovrd=off  block_type=slice
  high32_1 : xbsIndex_r4/Slice  nbits=32  boolean_output=off  mode=Lower Bit Location + Width  bit1=-31  base1=MSB of Input  bit0=32  base0=LSB of Input  dbl_ovrd=off  block_type=slice
  low32_ : xbsIndex_r4/Slice  nbits=32  boolean_output=off  mode=Lower Bit Location + Width  bit1=-31  base1=MSB of Input  bit0=0  base0=LSB of Input  dbl_ovrd=off  block_type=slice
  low32_1 : xbsIndex_r4/Slice  nbits=32  boolean_output=off  mode=Lower Bit Location + Width  bit1=-31  base1=MSB of Input  bit0=0  base0=LSB of Input  dbl_ovrd=off  block_type=slice
  ValidPulse : Outport
  ImagOutRawLo : Outport  Port=2
  RealOutRawLo : Outport  Port=3
  ValiidFlag : Outport  Port=4
  ImagOutRawHi : Outport  Port=5
  RealOutRawHi : Outport  Port=6
  wires:
  SFix34_32_1/1 -> SFix64_32_1/1
  Relational/1 -> Logical2/1, Logical1/2, Logical1/1, Gateway Out6/1, Logical/2
  Counter32_/1 -> Gateway Out1/1, Relational/2
  [winddata] -> SFix34_32_1/1, Gateway Out13/1, SFix34_32_0/1
  CosIn/1 -> SFix34_32_1/2
  DFTLen/1 -> Relational/1
  ValidIn/1 -> Logical2/2, Gateway Out9/1, Delay2/1
  Clear/1 -> Accumulator2/2, Gateway Out7/1, Accumulator1/2, Accumulator/2, Counter32_/1
  SinIn/1 -> Gateway Out12/1, SFix34_32_0/2
  Logical/1 -> Delay/1
  Delay/1 -> Accumulator1/3, Accumulator/3
  Logical1/1 -> Delay1/1
  Delay1/1 -> Gateway Out8/1, ValiidFlag/1, edge_detect/1
  edge_detect/1 -> Gateway Out10/1, ValidPulse/1
  Gateway Out6/1 -> Scope8/2
  Gateway Out7/1 -> Scope8/3
  Gateway Out8/1 -> Scope8/1
  Gateway Out9/1 -> Scope8/4
  Gateway Out10/1 -> Scope8/5
  Gateway Out1/1 -> Scope8/6
  Logical2/1 -> Accumulator2/3, Counter32_/2
  Delay2/1 -> Logical/1
  SFix34_32_0/1 -> SFix64_32_/1
  Gateway Out2/1 -> dftsignals/1
  Gateway Out3/1 -> dftsignals/2
  Gateway Out5/1 -> dftsignals/3
  Gateway Out13/1 -> dftsignals/5
  Gateway Out11/1 -> dftsignals/4
  Gateway Out12/1 -> dftsignals/6
  SFix64_32_/1 -> Gateway Out5/1, Accumulator1/1
  SFix64_32_1/1 -> Gateway Out11/1, Accumulator/1
  Accumulator1/1 -> Gateway Out2/1, high32_/1, low32_/1
  Accumulator/1 -> high32_1/1, low32_1/1, Gateway Out3/1
  low32_/1 -> Gateway Out4/1, ImagOutRawLo/1
  high32_/1 -> Gateway Out14/1, ImagOutRawHi/1
  low32_1/1 -> Gateway Out15/1, RealOutRawLo/1
  high32_1/1 -> Gateway Out16/1, RealOutRawHi/1
  Gateway Out15/1 -> dftouts/3
  Gateway Out16/1 -> dftouts/4
  Gateway Out14/1 -> dftouts/2
  Gateway Out4/1 -> dftouts/1
  ROM/1 -> Gateway Out18/1, Mult/1
  Delay3/1 -> Mult/2
  Mult/1 -> Gateway Out17/1, [winddata]
  Top6_/1 -> Gateway Out19/1, ROM/1
  Accumulator2/1 -> Gateway Out20/1, Top6_/1
  SixFourDivLen/1 -> Accumulator2/1
  DataIn/1 -> Gateway Out21/1, Delay3/1
  Gateway Out17/1 -> dftouts1/1
  Gateway Out18/1 -> dftouts1/2
  Gateway Out19/1 -> dftouts1/3
  Gateway Out20/1 -> dftouts1/4
  Gateway Out21/1 -> dftouts1/5

== system networkanalyzer/FreqSweeper ==
  startFreq : Inport
  endFreq : Inport  Port=2
  incFreq : Inport  Port=3
  fregAddend : Inport  Port=4
  rstFreq : Inport  Port=5
  Accumulator : xbsIndex_r4/Accumulator  operation=Add  n_bits=32  overflow=Wrap  scale=1  rst=on  hasbypass=off  en=on  dbl_ovrd=off  use_behavioral_HDL=on  implementation=Fabric  block_type=accum
  AddSub : xbsIndex_r4/AddSub  mode=Addition  use_carryin=off  use_carryout=off  en=off  latency=0  precision=User Defined  arith_type=Unsigned  n_bits=32  bin_pt=0  quantization=Truncate  overflow=Wrap  dbl_ovrd=off  use_behavioral_HDL=off  hw_selection=Fabric  pipelined=off  block_type=addsub
  Relational : xbsIndex_r4/Relational  mode=a<b  en=off  latency=0  dbl_ovrd=off  block_type=relational
  outFreq : Outport
  isLastFreq : Outport  Port=2
  wires:
  endFreq/1 -> Relational/1
  fregAddend/1 -> Accumulator/1
  Accumulator/1 -> AddSub/1
  incFreq/1 -> Accumulator/3
  startFreq/1 -> AddSub/2
  AddSub/1 -> outFreq/1, Relational/2
  rstFreq/1 -> Accumulator/2
  Relational/1 -> isLastFreq/1

== system networkanalyzer/LO_SLE ==
  sim_reg : Inport
  io_delay : xbsIndex_r4/Delay  rst=off  infoeditControl=Selection of Reset will increase slice count due to use of real FFs and instead of SRLs  en=off  latency=0  dbl_ovrd=off  reg_retiming=on  block_type=delay
  networkanalyzer_LO_SLE_user_data_out : xbsIndex_r4/Gateway In  gui_display_data_type=Fixed-point  arith_type=Unsigned  n_bits=32  bin_pt=0  preci_type=Single  exp_width=8  frac_width=24  quantization="Round  (unbiased: +/- Inf)"  overflow=Saturate  period=1  dbl_ovrd=off  timing_constraint=None  locs_specified=off  LOCs={}  UseAsADC=off  ADCChannel='1'  inherit_from_input=off  hdl_port=on  block_type=gatewayin
  reint1 : xbsIndex_r4/Reinterpret  force_arith_type=on  arith_type=Unsigned  force_bin_pt=on  bin_pt=0  block_type=reinterpret
  slice_reg : xbsIndex_r4/Slice  nbits=32  boolean_output=off  mode=Lower Bit Location + Width  bit1=0  base1=MSB of Input  bit0=0  base0=LSB of Input  dbl_ovrd=off  block_type=slice
  in_reg : Outport
  wires:
  networkanalyzer_LO_SLE_user_data_out/1 -> io_delay/1
  sim_reg/1 -> networkanalyzer_LO_SLE_user_data_out/1
  io_delay/1 -> slice_reg/1
  slice_reg/1 -> reint1/1
  reint1/1 -> in_reg/1

== system networkanalyzer/SER_DI ==
  sim_reg : Inport
  io_delay : xbsIndex_r4/Delay  rst=off  infoeditControl=Selection of Reset will increase slice count due to use of real FFs and instead of SRLs  en=off  latency=0  dbl_ovrd=off  reg_retiming=on  block_type=delay
  networkanalyzer_SER_DI_user_data_out : xbsIndex_r4/Gateway In  gui_display_data_type=Fixed-point  arith_type=Unsigned  n_bits=32  bin_pt=0  preci_type=Single  exp_width=8  frac_width=24  quantization="Round  (unbiased: +/- Inf)"  overflow=Saturate  period=1  dbl_ovrd=off  timing_constraint=None  locs_specified=off  LOCs={}  UseAsADC=off  ADCChannel='1'  inherit_from_input=off  hdl_port=on  block_type=gatewayin
  reint1 : xbsIndex_r4/Reinterpret  force_arith_type=on  arith_type=Unsigned  force_bin_pt=on  bin_pt=0  block_type=reinterpret
  slice_reg : xbsIndex_r4/Slice  nbits=32  boolean_output=off  mode=Lower Bit Location + Width  bit1=0  base1=MSB of Input  bit0=0  base0=LSB of Input  dbl_ovrd=off  block_type=slice
  in_reg : Outport
  wires:
  networkanalyzer_SER_DI_user_data_out/1 -> io_delay/1
  sim_reg/1 -> networkanalyzer_SER_DI_user_data_out/1
  io_delay/1 -> slice_reg/1
  slice_reg/1 -> reint1/1
  reint1/1 -> in_reg/1

== system networkanalyzer/SWAT_LE ==
  sim_reg : Inport
  io_delay : xbsIndex_r4/Delay  rst=off  infoeditControl=Selection of Reset will increase slice count due to use of real FFs and instead of SRLs  en=off  latency=0  dbl_ovrd=off  reg_retiming=on  block_type=delay
  networkanalyzer_SWAT_LE_user_data_out : xbsIndex_r4/Gateway In  gui_display_data_type=Fixed-point  arith_type=Unsigned  n_bits=32  bin_pt=0  preci_type=Single  exp_width=8  frac_width=24  quantization="Round  (unbiased: +/- Inf)"  overflow=Saturate  period=1  dbl_ovrd=off  timing_constraint=None  locs_specified=off  LOCs={}  UseAsADC=off  ADCChannel='1'  inherit_from_input=off  hdl_port=on  block_type=gatewayin
  reint1 : xbsIndex_r4/Reinterpret  force_arith_type=on  arith_type=Unsigned  force_bin_pt=on  bin_pt=0  block_type=reinterpret
  slice_reg : xbsIndex_r4/Slice  nbits=32  boolean_output=off  mode=Lower Bit Location + Width  bit1=0  base1=MSB of Input  bit0=0  base0=LSB of Input  dbl_ovrd=off  block_type=slice
  in_reg : Outport
  wires:
  networkanalyzer_SWAT_LE_user_data_out/1 -> io_delay/1
  sim_reg/1 -> networkanalyzer_SWAT_LE_user_data_out/1
  io_delay/1 -> slice_reg/1
  slice_reg/1 -> reint1/1
  reint1/1 -> in_reg/1

== system networkanalyzer/SixFourDivLen32p26 ==
  sim_reg : Inport
  io_delay : xbsIndex_r4/Delay  rst=off  infoeditControl=Selection of Reset will increase slice count due to use of real FFs and instead of SRLs  en=off  latency=0  dbl_ovrd=off  reg_retiming=on  block_type=delay
  networkanalyzer_SixFourDivLen32p26_user_data_out : xbsIndex_r4/Gateway In  gui_display_data_type=Fixed-point  arith_type=Unsigned  n_bits=32  bin_pt=0  preci_type=Single  exp_width=8  frac_width=24  quantization="Round  (unbiased: +/- Inf)"  overflow=Saturate  period=1  dbl_ovrd=off  timing_constraint=None  locs_specified=off  LOCs={}  UseAsADC=off  ADCChannel='1'  inherit_from_input=off  hdl_port=on  block_type=gatewayin
  reint1 : xbsIndex_r4/Reinterpret  force_arith_type=on  arith_type=Unsigned  force_bin_pt=on  bin_pt=0  block_type=reinterpret
  slice_reg : xbsIndex_r4/Slice  nbits=32  boolean_output=off  mode=Lower Bit Location + Width  bit1=0  base1=MSB of Input  bit0=0  base0=LSB of Input  dbl_ovrd=off  block_type=slice
  in_reg : Outport
  wires:
  networkanalyzer_SixFourDivLen32p26_user_data_out/1 -> io_delay/1
  sim_reg/1 -> networkanalyzer_SixFourDivLen32p26_user_data_out/1
  io_delay/1 -> slice_reg/1
  slice_reg/1 -> reint1/1
  reint1/1 -> in_reg/1

== system networkanalyzer/Stack4_ ==
  note: To Push to stack
      | Setdata in on clk0
      | Push =1 on clk0
      | Push=0 on clk1
      | This does a push
      | After push, addr has been incremented.
      |
      | Pop on clk 0, which decs address
      | read whatever is on Dataout on clk1
  dataIn : Inport
  Push : Inport  Port=2
  Pop : Inport  Port=3
  Rst : Inport  Port=4
  Gateway Out{1..5,7} (6 alike) : xbsIndex_r4/Gateway Out  inherit_from_input=off  hdl_port=off  timing_constraint=None  locs_specified=off  LOCs={}  UseAsDAC=off  DACChannel='1'  block_type=gatewayout
  Mux : xbsIndex_r4/Mux  inputs=4  en=off  latency=0  precision=Full  arith_type=Unsigned  n_bits=16  bin_pt=14  quantization=Truncate  overflow=Wrap  dbl_ovrd=off  block_type=mux
  RegAddr : Subsystem
  RegAddr1 : Subsystem
  RegAddr2 : Subsystem
  RegAddr3 : Subsystem
  Scope1 : Scope  NumInputPorts=8
      settings: YMin=0~-5~-5~-5~-5~-5~-5~-5  YMax=300000~5~5~5~5~5~5~5  SaveName=ScopeData11  MaxDataPoints=10000
  updownCnt : Subsystem
  DataOut : Outport
  wires:
  dataIn/1 -> Gateway Out3/1, RegAddr3/1(Data), RegAddr1/1(Data), RegAddr/1(Data), RegAddr2/1(Data)
  updownCnt/1(Out) -> Gateway Out4/1, Mux/1, RegAddr1/2(Addr), RegAddr/2(Addr), RegAddr2/2(Addr), RegAddr3/2(Addr)
  Pop/1 -> Gateway Out1/1, updownCnt/1(Dec)
  Push/1 -> Gateway Out7/1, RegAddr3/3(WE), RegAddr1/3(WE), RegAddr/3(WE), RegAddr2/3(WE), updownCnt/2(Inc)
  Rst/1 -> Gateway Out2/1, updownCnt/3(Rst)
  RegAddr3/1(DataOut) -> Mux/5
  RegAddr1/1(DataOut) -> Mux/4
  Mux/1 -> Gateway Out5/1, DataOut/1
  RegAddr/1(DataOut) -> Mux/3
  RegAddr2/1(DataOut) -> Mux/2
  Gateway Out7/1 -> Scope1/1
  Gateway Out1/1 -> Scope1/2
  Gateway Out2/1 -> Scope1/3
  Gateway Out3/1 -> Scope1/4
  Gateway Out4/1 -> Scope1/5
  Gateway Out5/1 -> Scope1/6

== system networkanalyzer/adcWaveMem ==
  Start : Inport
  Sel : Inport  Port=2
  Src0 : Inport  Port=3
  Src1 : Inport  Port=4
  WE : Inport  Port=5
  WE1 : Inport  Port=6
  Logical : xbsIndex_r4/Logical  logical_function=OR  inputs=2  en=off  latency=0  precision=Full  arith_type=Unsigned  n_bits=16  bin_pt=0  align_bp=on  dbl_ovrd=off  block_type=logical
  MemRecord : Subsystem
  Mux : xbsIndex_r4/Mux  inputs=2  en=off  latency=0  precision=Full  arith_type=Unsigned  n_bits=16  bin_pt=14  quantization=Truncate  overflow=Wrap  dbl_ovrd=off  block_type=mux
  Slice : xbsIndex_r4/Slice  nbits=12  boolean_output=off  mode=Lower Bit Location + Width  bit1=0  base1=LSB of Input  bit0=0  base0=LSB of Input  dbl_ovrd=off  block_type=slice
  edge_detect : casper_library_misc/edge_detect  edge=Rising  polarity=Active High  x_in=[0 0.08 0.08 0.16 0.16 0.24 0.24 0.32 0.32 0.4]  y_in="[-1 -1  1  1  1  1  1  1  1  1]"  x_out=[0.6 0.68 0.68 0.76 0.76 0.84 0.84 0.92 0.92 1]  y_out="[-1 -1  1  1 -1 -1 -1 -1 -1 -1]"
  Out1 : Outport
  wires:
  Sel/1 -> Mux/1
  edge_detect/1 -> Logical/2
  WE/1 -> Logical/1
  Src0/1 -> Mux/2
  Src1/1 -> Mux/3
  WE1/1 -> edge_detect/1
  MemRecord/1(memDone) -> Out1/1
  Start/1 -> MemRecord/1(Start)
  Logical/1 -> MemRecord/3(WE)
  Slice/1 -> MemRecord/2(DataIn)
  Mux/1 -> Slice/1

== system networkanalyzer/adcWaveMem1 ==
  Start : Inport
  Sel : Inport  Port=2
  Src0 : Inport  Port=3
  Src1 : Inport  Port=4
  WE : Inport  Port=5
  WE1 : Inport  Port=6
  Logical : xbsIndex_r4/Logical  logical_function=OR  inputs=2  en=off  latency=0  precision=Full  arith_type=Unsigned  n_bits=16  bin_pt=0  align_bp=on  dbl_ovrd=off  block_type=logical
  MemRecord : Subsystem
  Mux : xbsIndex_r4/Mux  inputs=2  en=off  latency=0  precision=Full  arith_type=Unsigned  n_bits=16  bin_pt=14  quantization=Truncate  overflow=Wrap  dbl_ovrd=off  block_type=mux
  Slice : xbsIndex_r4/Slice  nbits=12  boolean_output=off  mode=Lower Bit Location + Width  bit1=0  base1=LSB of Input  bit0=0  base0=LSB of Input  dbl_ovrd=off  block_type=slice
  edge_detect : casper_library_misc/edge_detect  edge=Rising  polarity=Active High  x_in=[0 0.08 0.08 0.16 0.16 0.24 0.24 0.32 0.32 0.4]  y_in="[-1 -1  1  1  1  1  1  1  1  1]"  x_out=[0.6 0.68 0.68 0.76 0.76 0.84 0.84 0.92 0.92 1]  y_out="[-1 -1  1  1 -1 -1 -1 -1 -1 -1]"
  Out1 : Outport
  wires:
  Sel/1 -> Mux/1
  edge_detect/1 -> Logical/2
  WE/1 -> Logical/1
  Src0/1 -> Mux/2
  Src1/1 -> Mux/3
  WE1/1 -> edge_detect/1
  MemRecord/1(memDone) -> Out1/1
  Start/1 -> MemRecord/1(Start)
  Logical/1 -> MemRecord/3(WE)
  Slice/1 -> MemRecord/2(DataIn)
  Mux/1 -> Slice/1

== system networkanalyzer/adcWaveMem2 ==
  Start : Inport
  Sel : Inport  Port=2
  Src0 : Inport  Port=3
  Src1 : Inport  Port=4
  WE : Inport  Port=5
  WE1 : Inport  Port=6
  Logical : xbsIndex_r4/Logical  logical_function=OR  inputs=2  en=off  latency=0  precision=Full  arith_type=Unsigned  n_bits=16  bin_pt=0  align_bp=on  dbl_ovrd=off  block_type=logical
  MemRecord : Subsystem
  Mux : xbsIndex_r4/Mux  inputs=2  en=off  latency=0  precision=Full  arith_type=Unsigned  n_bits=16  bin_pt=14  quantization=Truncate  overflow=Wrap  dbl_ovrd=off  block_type=mux
  Slice : xbsIndex_r4/Slice  nbits=12  boolean_output=off  mode=Lower Bit Location + Width  bit1=0  base1=LSB of Input  bit0=0  base0=LSB of Input  dbl_ovrd=off  block_type=slice
  edge_detect : casper_library_misc/edge_detect  edge=Rising  polarity=Active High  x_in=[0 0.08 0.08 0.16 0.16 0.24 0.24 0.32 0.32 0.4]  y_in="[-1 -1  1  1  1  1  1  1  1  1]"  x_out=[0.6 0.68 0.68 0.76 0.76 0.84 0.84 0.92 0.92 1]  y_out="[-1 -1  1  1 -1 -1 -1 -1 -1 -1]"
  Out1 : Outport
  wires:
  Sel/1 -> Mux/1
  edge_detect/1 -> Logical/2
  WE/1 -> Logical/1
  Src0/1 -> Mux/2
  Src1/1 -> Mux/3
  WE1/1 -> edge_detect/1
  MemRecord/1(memDone) -> Out1/1
  Start/1 -> MemRecord/1(Start)
  Logical/1 -> MemRecord/3(WE)
  Slice/1 -> MemRecord/2(DataIn)
  Mux/1 -> Slice/1
